simulink model "untitled"  (R2022a)
settings: Solver=VariableStepAuto  StartTime=0.0  StopTime=10.0  RelTol=1e-3
undefined symbols (not defined in the file): robotXDragCoefficients, robotYDragCoefficients, robotZDragCoefficients
settings Model: Creator=hollis  LastModifiedBy=hollis

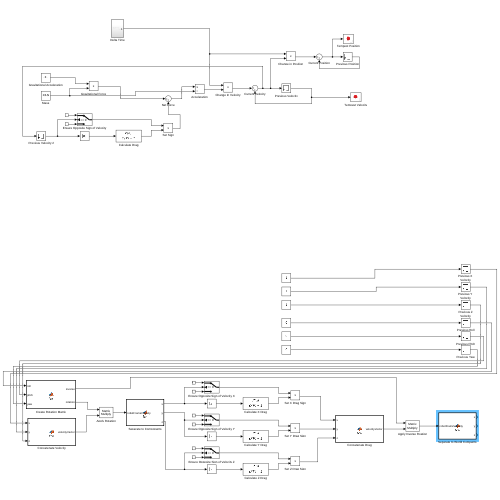
[thumbnail: Simulink's stored preview of the top-level diagram]
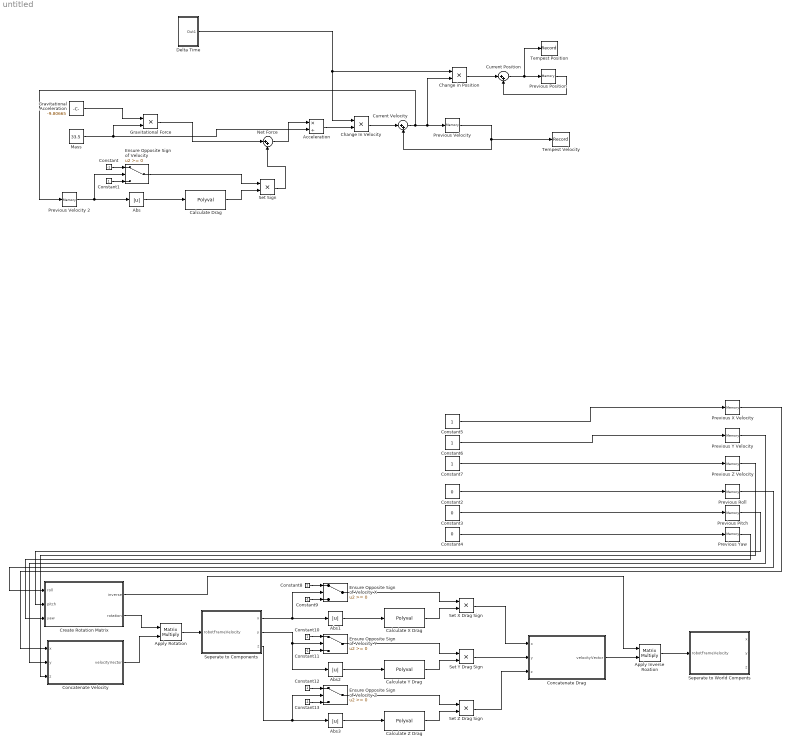
== system untitled ==
  Abs{,1..3} (4 alike) : Abs  SaturateOnIntegerOverflow=off
  Acceleration : Product  Inputs=*/
  Apply Inverse Roation : Product  Multiplication=Matrix(*)
  Apply Rotation : Product  Multiplication=Matrix(*)
  Calculate Drag : Polyval  Coefs=[460, 35, 0]
  Calculate X Drag : Polyval  Coefs=robotXDragCoefficients
  Calculate Y Drag : Polyval  Coefs=robotYDragCoefficients
  Calculate Z Drag : Polyval  Coefs=robotZDragCoefficients
  Change In Velocity : Product
  Change in Position : Product
  Concatenate Drag : MATLAB Function  TreatAsAtomicUnit=on
  Concatenate Velocity : MATLAB Function  TreatAsAtomicUnit=on
  Constant{,9,11,13} (4 alike) : Constant  Value=-1
  Constant{1,5..8,10,12} (7 alike) : Constant
  Constant2 : Constant  Value=0
  Constant3 : Constant  Value=0
  Constant4 : Constant  Value=0
  Create Rotation Matrix : MATLAB Function  TreatAsAtomicUnit=on
  Current Position : Sum  Inputs=|++
  Current Velocity : Sum  Inputs=|++
  Delta Time : Subsystem
  Ensure Opposite Sign of Velocity : Switch  SaturateOnIntegerOverflow=off  InputSameDT=off
  Ensure Opposite Sign of Velocity X : Switch  SaturateOnIntegerOverflow=off  InputSameDT=off
  Ensure Opposite Sign of Velocity Y : Switch  SaturateOnIntegerOverflow=off  InputSameDT=off
  Ensure Opposite Sign of Velocity Z : Switch  SaturateOnIntegerOverflow=off  InputSameDT=off
  Gravitational Acceleration : Constant  Value=-9.80665
  Gravitational Force : Product
  Mass : Constant  Value=33.5
  Net Force : Sum  Inputs=|++
  Previous Pitch : Memory
  Previous Position : Memory
  Previous Roll : Memory
  Previous Velocity : Memory
  Previous Velocity 2 : Memory
  Previous X Velocity : Memory
  Previous Y Velocity : Memory
  Previous Yaw : Memory
  Previous Z Velocity : Memory
  Seperate to Components : MATLAB Function  TreatAsAtomicUnit=on
  Seperate to World Compents : MATLAB Function  TreatAsAtomicUnit=on
  Set Sign : Product
  Set X Drag Sign : Product
  Set Y Drag Sign : Product
  Set Z Drag Sign : Product
  Tempest Position : Record  FileSettingsInternal="{\"entries\":[{\"content\":{\"excelSettings\":{\"content\":{},\"type\":\"Streamout.ExcelSettings\"}},\"type\":\"Streamout.FileSettingStorage\",\"uuid\":\"199525da-55ae-4564-878d-6915dab59d0a\"}],\"packageUris\":[\"http://schema.mathworks.com/mf0/streamout_blocks/R2020a\"],\"version\":\"1.0\"}"  SignalsInternal="{\"entries\":[{\"content\":{\"signals\":[{\"content\":{\"blockPath\":[\"untitled/Tempest Position\"],\"channel\":[],\"dimensions\":[1],\"domain\":\"untitled/Tempest Position\",\"lineColor\":\"#d95319\",\"plots\":[1],\"port\":1,\"sid\":[\"\"],\"signalID\":189,\"signalName\":\"Current Position\"},\"type\":\"RecordBlkView.Signal\",\"uuid\":\"d74b57f0-48a2-46c2-86c0-f61d41647e8b\"}]},\"type\":\"RecordBlkView.InputSignals\",\"uuid\":\"b0b27219-34df-4c19-9ac4-1c882c491d06\"}],\"packageUris\":[\"http://schema.mathworks.com/mf0/streamout_blocks/R2020a\"],\"version\":\"1.0\"}"  VisualizationBindings="{\"sparklinesplugin\":{\"info\":[{\"bindingParametersList\":[],\"subplotID\":1}]}}"
  Tempest Velocity : Record  FileSettingsInternal="{\"entries\":[{\"content\":{\"excelSettings\":{\"content\":{},\"type\":\"Streamout.ExcelSettings\"}},\"type\":\"Streamout.FileSettingStorage\",\"uuid\":\"7598b46f-fc40-4f35-ab8a-c3cd655a6376\"}],\"packageUris\":[\"http://schema.mathworks.com/mf0/streamout_blocks/R2020a\"],\"version\":\"1.0\"}"  SignalsInternal="{\"entries\":[{\"content\":{\"signals\":[{\"content\":{\"blockPath\":[\"untitled/Tempest Velocity\"],\"channel\":[],\"dimensions\":[1],\"domain\":\"untitled/Tempest Velocity\",\"lineColor\":\"#edb120\",\"plots\":[1],\"port\":1,\"sid\":[\"\"],\"signalID\":193,\"signalName\":\"Previous Velocity\"},\"type\":\"RecordBlkView.Signal\",\"uuid\":\"9ce42202-10ae-455a-a906-496b26bdc8e9\"}]},\"type\":\"RecordBlkView.InputSignals\",\"uuid\":\"f0455b54-dcc6-47df-96b6-3eed90f76b3d\"}],\"packageUris\":[\"http://schema.mathworks.com/mf0/streamout_blocks/R2020a\"],\"version\":\"1.0\"}"  VisualizationBindings="{\"sparklinesplugin\":{\"info\":[{\"bindingParametersList\":[],\"subplotID\":1}]}}"
  wires:
  Net Force/1 -> Acceleration/1
  Gravitational Force/1 -> Net Force/1
  Set Sign/1 -> Net Force/2
  Calculate Drag/1 -> Set Sign/2
  Change in Position/1 -> Current Position/1
  Current Position/1 -> Tempest Position/1, Previous Position/1
  Previous Velocity/1 -> Current Velocity/2, Tempest Velocity/1
  Gravitational Acceleration/1 -> Gravitational Force/1
  Mass/1 -> Acceleration/2, Gravitational Force/2
  Constant1/1 -> Ensure Opposite Sign of Velocity/3
  Abs/1 -> Calculate Drag/1
  Current Velocity/1 -> Previous Velocity 2/1, Change in Position/2, Previous Velocity/1
  Change In Velocity/1 -> Current Velocity/1
  Previous Velocity 2/1 -> Abs/1, Ensure Opposite Sign of Velocity/2
  Constant/1 -> Ensure Opposite Sign of Velocity/1
  Previous Position/1 -> Current Position/2
  Ensure Opposite Sign of Velocity/1 -> Set Sign/1
  Acceleration/1 -> Change In Velocity/2
  Delta Time/1(Out1) -> Change In Velocity/1, Change in Position/1
  Previous Roll/1 -> Create Rotation Matrix/1(roll)
  Previous Pitch/1 -> Create Rotation Matrix/2(pitch)
  Previous Yaw/1 -> Create Rotation Matrix/3(yaw)
  Previous Z Velocity/1 -> Concatenate Velocity/3(z)
  Previous Y Velocity/1 -> Concatenate Velocity/2(y)
  Previous X Velocity/1 -> Concatenate Velocity/1(x)
  Create Rotation Matrix/2(rotation) -> Apply Rotation/1
  Concatenate Velocity/1(velocityVector) -> Apply Rotation/2
  Constant4/1 -> Previous Yaw/1
  Constant3/1 -> Previous Pitch/1
  Constant2/1 -> Previous Roll/1
  Constant5/1 -> Previous X Velocity/1
  Constant6/1 -> Previous Y Velocity/1
  Constant7/1 -> Previous Z Velocity/1
  Apply Rotation/1 -> Seperate to Components/1(robotFrameVelocity)
  Abs1/1 -> Calculate X Drag/1
  Ensure Opposite Sign of Velocity X/1 -> Set X Drag Sign/1
  Constant9/1 -> Ensure Opposite Sign of Velocity X/3
  Constant8/1 -> Ensure Opposite Sign of Velocity X/1
  Calculate X Drag/1 -> Set X Drag Sign/2
  Seperate to Components/1(x) -> Abs1/1, Ensure Opposite Sign of Velocity X/2
  Seperate to Components/2(y) -> Abs2/1, Ensure Opposite Sign of Velocity Y/2
  Ensure Opposite Sign of Velocity Y/1 -> Set Y Drag Sign/1
  Constant11/1 -> Ensure Opposite Sign of Velocity Y/3
  Constant10/1 -> Ensure Opposite Sign of Velocity Y/1
  Calculate Y Drag/1 -> Set Y Drag Sign/2
  Abs2/1 -> Calculate Y Drag/1
  Seperate to Components/3(z) -> Abs3/1, Ensure Opposite Sign of Velocity Z/2
  Ensure Opposite Sign of Velocity Z/1 -> Set Z Drag Sign/1
  Constant13/1 -> Ensure Opposite Sign of Velocity Z/3
  Constant12/1 -> Ensure Opposite Sign of Velocity Z/1
  Calculate Z Drag/1 -> Set Z Drag Sign/2
  Abs3/1 -> Calculate Z Drag/1
  Create Rotation Matrix/1(inverse) -> Apply Inverse Roation/1
  Set X Drag Sign/1 -> Concatenate Drag/1(x)
  Set Y Drag Sign/1 -> Concatenate Drag/2(y)
  Set Z Drag Sign/1 -> Concatenate Drag/3(z)
  Concatenate Drag/1(velocityVector) -> Apply Inverse Roation/2
  Apply Inverse Roation/1 -> Seperate to World Compents/1(robotFrameVelocity)

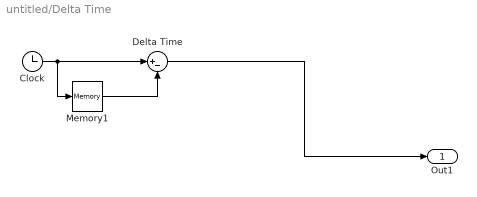
== system untitled/Delta Time ==
  Clock : Clock
  Delta Time : Sum  Inputs=|+-
  Memory1 : Memory
  Out1 : Outport
  wires:
  Memory1/1 -> Delta Time/2
  Clock/1 -> Memory1/1, Delta Time/1
  Delta Time/1 -> Out1/1

== matlab function untitled/Concatenate Velocity ==
  data: x input; velocityVector output; y input; z input
function velocityVector = fcn(x,y,z)

velocityVector = [x; y; z];

== matlab function untitled/Create Rotation Matrix ==
  data: inverse output; roll input; rotation output; pitch input; yaw input
function [inverse, rotation] = fcn(roll, pitch, yaw)

y = [yaw, pitch, roll];


rotation = eul2rotm(y);
inverse = inv(rotation);

== matlab function untitled/Seperate to Components ==
  data: x output; robotFrameVelocity input; y output; z output
function [x, y, z] = fcn(robotFrameVelocity)

x = robotFrameVelocity(1, 1);
y = robotFrameVelocity(2, 1);
z = robotFrameVelocity(3, 1);

== matlab function untitled/Concatenate Drag ==
  data: x input; velocityVector output; y input; z input
function velocityVector = fcn(x,y,z)

velocityVector = [x; y; z];

== matlab function untitled/Seperate to World Compents ==
  data: x output; robotFrameVelocity input; y output; z output
function [x, y, z] = fcn(robotFrameVelocity)

x = robotFrameVelocity(1, 1);
y = robotFrameVelocity(2, 1);
z = robotFrameVelocity(3, 1);
